simulink model "resolucion_sim_ej_4e_final_31_07_2023"  (R2018b)
settings: Solver=ode4  StartTime=0.0  StopTime=300  FixedStep=0.0001  RelTol=1e-3
values from neighbouring files (symbols this model uses):
  u0 = 2    [ejercicio4.m]
  x0 = [9 5 4]    [ejercicio4.m]
  y0 = 2    [ejercicio4.m]
libraries: cstblocks x1
settings Model: Creator=aghersin  LastModifiedBy=zambr
settings OptimizationCC: LifeSpan=inf
settings DebuggingCC: SFExecutionAtInitializationDiag=none
settings SFSimCC: SimUseLocalCustomCode=off
settings RTWCC: RTWUseLocalCustomCode=off
settings CodeAppCC: StateflowObjectComments=on

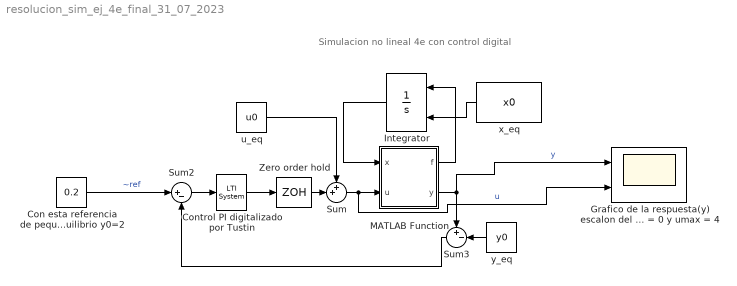
== system resolucion_sim_ej_4e_final_31_07_2023 ==
  note: Simulacion no lineal 4e con control digital
  "Con esta referencia de pequeña señal(20 %), quiero que en la salida y se mueva un 20% con respecto al equilibrio y0=2" : Constant  Value=0.2
  Control PI digitalizado por Tustin : cstblocks/LTI System  sys=Cd  IC=[]
  "Grafico de la respuesta(y) escalon del sistema ante la referencia de pequeña señal 0.2, en que la salida se mueve un 20% con respecto al equilibrio y0=2. Despues se grafica acción de control u que es la respuesta al escalon a la referencia de pequeña señal ~ref=0.2, donde se puede ver que u no se excede entre los limites umin = 0 y umax = 4" : Scope  NumInputPorts=2
  Integrator : Integrator  InitialConditionSource=external
  MATLAB Function : MATLAB Function  TreatAsAtomicUnit=on
  Sum : Sum  Inputs=++|
  Sum2 : Sum  Inputs=|+-
  Sum3 : Sum  Inputs=+-|
  Zero order hold : ZeroOrderHold  SampleTime=-1
  u_eq : Constant  Value=u0
  x_eq : Constant  Value=x0
  y_eq : Constant  Value=y0
  wires:
  Integrator/1 -> MATLAB Function/1(x)
  MATLAB Function/1(f) -> Integrator/1
  x_eq/1 -> Integrator/2
  y_eq/1 -> Sum3/2
  u_eq/1 -> Sum/1
  Sum2/1 -> Control PI digitalizado por Tustin/1
  Sum3/1 -> Sum2/2
  Sum/1 -> "Grafico de la respuesta(y) escalon del sistema ante la referencia de pequeña señal 0.2, en que la salida se mueve un 20% con respecto al equilibrio y0=2. Despues se grafica acción de control u que es la respuesta al escalon a la referencia de pequeña señal ~ref=0.2, donde se puede ver que u no se excede entre los limites umin = 0 y umax = 4"/2, MATLAB Function/2(u)  "u"
  "Con esta referencia de pequeña señal(20 %), quiero que en la salida y se mueva un 20% con respecto al equilibrio y0=2"/1 -> Sum2/1  "~ref"
  MATLAB Function/2(y) -> "Grafico de la respuesta(y) escalon del sistema ante la referencia de pequeña señal 0.2, en que la salida se mueve un 20% con respecto al equilibrio y0=2. Despues se grafica acción de control u que es la respuesta al escalon a la referencia de pequeña señal ~ref=0.2, donde se puede ver que u no se excede entre los limites umin = 0 y umax = 4"/1, Sum3/1  "y"
  Control PI digitalizado por Tustin/1 -> Zero order hold/1
  Zero order hold/1 -> Sum/2

== matlab function resolucion_sim_ej_4e_final_31_07_2023/MATLAB Function ==
  data: x input; u input; f output; y output
function [f,y] = fcn(x,u)

% Valores buscados en papel
alfa=1;
beta=2;% Es datos

% Las ecuaciones de estados
h1 = -alfa * sqrt(x(1)-x(2)) + u;
h2 = alfa * sqrt(x(1)-x(2)) - beta * sqrt(x(2)-x(3));
h3 = beta * sqrt(x(2)-x(3)) - sqrt(x(3));

f=[h1;h2;h3];

y = sqrt(x(3));
